simulink model "Control_with_duty"  (R2021a)
settings: Solver=VariableStepAuto  StartTime=0.0  StopTime=10  RelTol=1e-3
values from neighbouring files (symbols this model uses):
  Calc_delay = 20e-6    (= 2e-05)    [Control.m]
  J = 0.00052*1000    (= 0.52)    [Control.m]
  Kf = 0.1*10    (= 1)    [Control.m]
  Ki = double(vpasolve(num(3)==Ki/Lq,Ki))    [Control.m]
  Kp = double(vpasolve(num(2)==Rq/Lq+Kp/Lq,Kp))    [Control.m]
  lambda = 0.032    [Control.m]
  Ld = Lq    (= 5.25e-05)    [Control.m]
  Lq = 0.0525*10^-3    (= 5.25e-05)    [Control.m]
  Rd = 0.013/2    (= 0.0065)    [Control.m]
  Rq = Rd    (= 0.0065)    [Control.m]
  Ts = 1/Fsw    (= 9.3808630394e-05)    [Control.m]
  Vbat = 14.4*4    (= 57.6)    [Control.m]
libraries: mcbcontrolslib x6
settings Model: Creator=jacob  LastModifiedBy=jacob

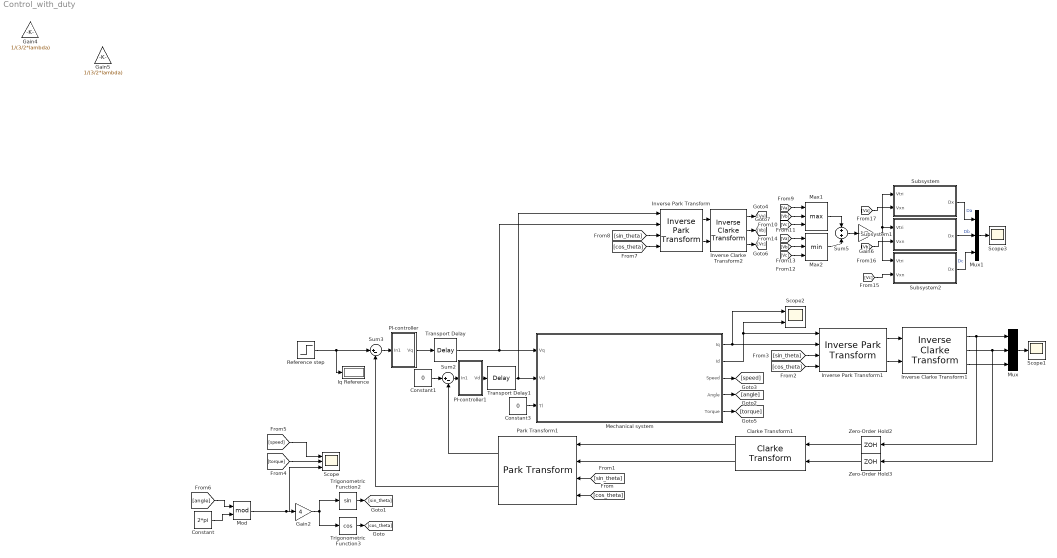
== system Control_with_duty ==
  Clarke Transform1 : mcbcontrolslib/Clarke Transform  VariantControl=Variant2
  Constant : Constant  Value=2*pi
  Constant1 : Constant  Value=0
  Constant3 : Constant  Value=0
  Gain2 : Gain  Gain=4
  Gain4 : Gain  Gain=1/(3/2*lambda)
  Gain5 : Gain  Gain=1/(3/2*lambda)
  Gain6 : Gain  Gain=-1/2
  Inverse Clarke Transform1 : mcbcontrolslib/Inverse Clarke Transform
      settings: SourceProductBaseCode=MT
  Inverse Clarke Transform2 : mcbcontrolslib/Inverse Clarke Transform
      settings: SourceProductBaseCode=MT
  Inverse Park Transform : mcbcontrolslib/Inverse Park Transform  AxisAlignment=D-axis
  Inverse Park Transform1 : mcbcontrolslib/Inverse Park Transform  AxisAlignment=D-axis
  Iq Reference : Display
      settings: Decimation=3
  Max1 : MinMax  Function=max  Inputs=3
  Max2 : MinMax  Inputs=3
  Mechanical system : Subsystem
  Mod : Math  Operator=mod  SaturateOnIntegerOverflow=on
  Mux : Mux  Inputs=3
  Mux1 : Mux  Inputs=3
  PI-controller : Subsystem
  PI-controller1 : Subsystem
  Park Transform1 : mcbcontrolslib/Park Transform  AxisAlignment=D-axis
      settings: SourceProductBaseCode=MT
  Reference step : Step  Time=0.1  After=311  SampleTime=0
  Scope : Scope  NumInputPorts=3
  Scope1 : Scope
  Scope2 : Scope  NumInputPorts=2
  Scope3 : Scope
  Subsystem : Subsystem
  Subsystem1 : Subsystem
  Subsystem2 : Subsystem
  Sum2 : Sum  Inputs=|+-
  Sum3 : Sum  Inputs=|+-
  Sum5 : Sum  Inputs=+|+
  Transport Delay : TransportDelay  DelayTime=Calc_delay
  Transport Delay1 : TransportDelay  DelayTime=Calc_delay
  Trigonometric Function2 : Trigonometry
  Trigonometric Function3 : Trigonometry  Operator=cos
  Zero-Order Hold2 : ZeroOrderHold  SampleTime=Ts
  Zero-Order Hold3 : ZeroOrderHold  SampleTime=Ts
  wires:
  Sum2/1 -> PI-controller1/1(In1)
  Inverse Park Transform1/2 -> Inverse Clarke Transform1/2
  [torque] -> Scope/2
  [sin_theta] -> Inverse Park Transform1/3
  [angle] -> Mod/1
  Constant/1 -> Mod/2
  Reference step/1 -> Sum3/1, Iq Reference/1
  Clarke Transform1/1 -> Park Transform1/1
  Clarke Transform1/2 -> Park Transform1/2
  Inverse Clarke Transform1/2 -> Zero-Order Hold3/1, Mux/2
  Inverse Park Transform1/1 -> Inverse Clarke Transform1/1
  Gain2/1 -> Trigonometric Function3/1, Trigonometric Function2/1
  Mux/1 -> Scope1/1
  Mechanical system/5(Torque) -> [torque]
  Sum3/1 -> PI-controller/1(In1)
  Inverse Clarke Transform1/3 -> Mux/3
  Park Transform1/1 -> Sum2/2
  Trigonometric Function3/1 -> [cos_theta]
  PI-controller1/1(Vd) -> Transport Delay1/1
  Mechanical system/1(Iq) -> Inverse Park Transform1/2, Scope2/1
  Inverse Clarke Transform1/1 -> Zero-Order Hold2/1, Mux/1
  Mechanical system/4(Angle) -> [angle]
  Mechanical system/2(Id) -> Inverse Park Transform1/1, Scope2/2
  Park Transform1/2 -> Sum3/2
  [cos_theta] -> Park Transform1/4
  [cos_theta] -> Inverse Park Transform1/4
  Constant3/1 -> Mechanical system/3(Tl)
  Mechanical system/3(Speed) -> [speed]
  Constant1/1 -> Sum2/1
  Zero-Order Hold3/1 -> Clarke Transform1/2
  [speed] -> Scope/1
  Mod/1 -> Scope/3, Gain2/1
  [sin_theta] -> Park Transform1/3
  PI-controller/1(Vq) -> Transport Delay/1
  Trigonometric Function2/1 -> [sin_theta]
  Zero-Order Hold2/1 -> Clarke Transform1/1
  Inverse Park Transform/1 -> Inverse Clarke Transform2/1
  Inverse Park Transform/2 -> Inverse Clarke Transform2/2
  [cos_theta] -> Inverse Park Transform/4
  [sin_theta] -> Inverse Park Transform/3
  Mux1/1 -> Scope3/1
  Subsystem/1(Dx) -> Mux1/1  "Da"
  Transport Delay1/1 -> Mechanical system/2(Vd), Inverse Park Transform/1
  Transport Delay/1 -> Inverse Park Transform/2, Mechanical system/1(Vq)
  Max2/1 -> Sum5/2
  Sum5/1 -> Gain6/1
  Max1/1 -> Sum5/1
  Inverse Clarke Transform2/1 -> [Va]
  Inverse Clarke Transform2/2 -> [Vb]
  Inverse Clarke Transform2/3 -> [Vc]
  Gain6/1 -> Subsystem1/1(Vtri), Subsystem/1(Vtri), Subsystem2/1(Vtri)
  [Va] -> Max2/1
  [Vb] -> Max2/2
  [Vc] -> Max2/3
  [Va] -> Max1/1
  [Vb] -> Max1/2
  [Vc] -> Max1/3
  [Va] -> Subsystem/2(Vxn)
  [Vc] -> Subsystem2/2(Vxn)
  [Vb] -> Subsystem1/2(Vxn)
  Subsystem2/1(Dx) -> Mux1/3  "Dc"
  Subsystem1/1(Dx) -> Mux1/2  "Db"

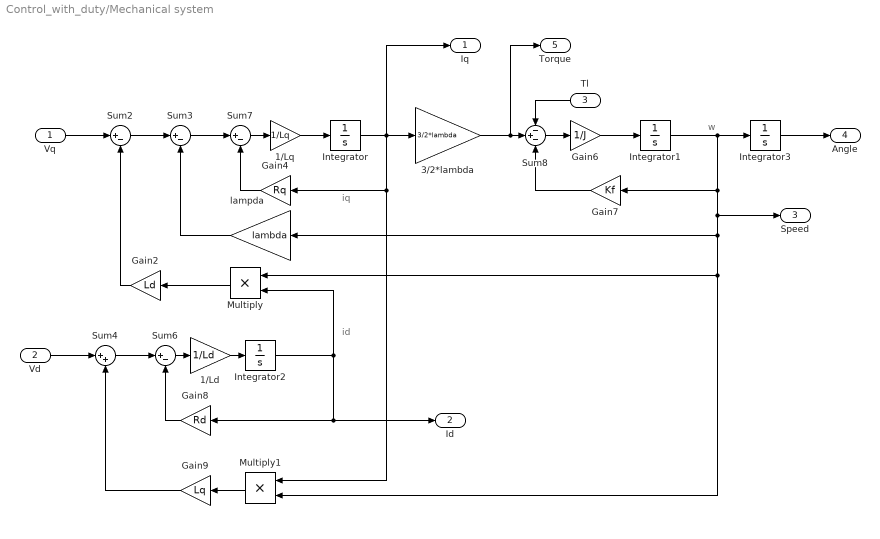
== system Control_with_duty/Mechanical system ==
  note: iq
  note: w
  note: id
  Vq : Inport
  Vd : Inport  Port=2
  Tl : Inport  Port=3
  1/Ld : Gain  Gain=1/Ld
  1/Lq : Gain  Gain=1/Lq
  3/2*lambda : Gain  Gain=3/2*lambda
  Gain2 : Gain  Gain=Ld
  Gain4 : Gain  Gain=Rq
  Gain6 : Gain  Gain=1/J
  Gain7 : Gain  Gain=Kf
  Gain8 : Gain  Gain=Rd
  Gain9 : Gain  Gain=Lq
  Integrator{,1..3} (4 alike) : Integrator
  Multiply : Product
  Multiply1 : Product
  Sum{2..3,6..7} (4 alike) : Sum  Inputs=|+-
  Sum4 : Sum  Inputs=|++
  Sum8 : Sum  Inputs=-+-
  lampda : Gain  Gain=lambda
  Iq : Outport
  Id : Outport  Port=2
  Speed : Outport  Port=3
  Angle : Outport  Port=4
  Torque : Outport  Port=5
  wires:
  Gain4/1 -> Sum7/2
  Sum2/1 -> Sum3/1
  Gain6/1 -> Integrator1/1
  Sum7/1 -> 1/Lq/1
  Vd/1 -> Sum4/1
  Sum6/1 -> 1/Ld/1
  Sum4/1 -> Sum6/1
  lampda/1 -> Sum3/2
  1/Lq/1 -> Integrator/1
  Gain2/1 -> Sum2/2
  Integrator2/1 -> Id/1, Gain8/1, Multiply/2
  Integrator1/1 -> Integrator3/1, Speed/1, Multiply1/2, Multiply/1, lampda/1, Gain7/1
  Sum8/1 -> Gain6/1
  Integrator/1 -> 3/2*lambda/1, Gain4/1, Multiply1/1, Iq/1
  Integrator3/1 -> Angle/1
  Multiply1/1 -> Gain9/1
  Gain9/1 -> Sum4/2
  Gain8/1 -> Sum6/2
  1/Ld/1 -> Integrator2/1
  Sum3/1 -> Sum7/1
  Multiply/1 -> Gain2/1
  Vq/1 -> Sum2/1
  3/2*lambda/1 -> Sum8/2, Torque/1
  Gain7/1 -> Sum8/3
  Tl/1 -> Sum8/1

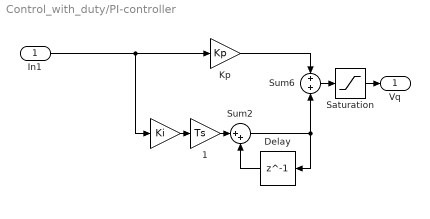
== system Control_with_duty/PI-controller ==
  In1 : Inport
  " " : Gain  Gain=Ki
  " 1" : Gain  Gain=Ts
  Delay : Delay  DelayLength=1  SampleTime=Ts
  Kp : Gain  Gain=Kp
  Saturation : Saturate  UpperLimit=Vbat  LowerLimit=-Vbat
  Sum2 : Sum  Inputs=|++
  Sum6 : Sum  Inputs=+|+
  Vq : Outport
  wires:
  " 1"/1 -> Sum2/1
  Delay/1 -> Sum2/2
  Kp/1 -> Sum6/1
  " "/1 -> " 1"/1
  Sum2/1 -> Delay/1, Sum6/2
  In1/1 -> " "/1, Kp/1
  Sum6/1 -> Saturation/1
  Saturation/1 -> Vq/1

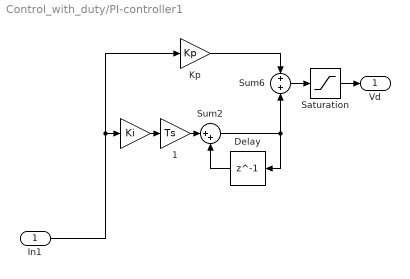
== system Control_with_duty/PI-controller1 ==
  In1 : Inport
  " " : Gain  Gain=Ki
  " 1" : Gain  Gain=Ts
  Delay : Delay  DelayLength=1  SampleTime=Ts
  Kp : Gain  Gain=Kp
  Saturation : Saturate  UpperLimit=Vbat  LowerLimit=-Vbat
  Sum2 : Sum  Inputs=|++
  Sum6 : Sum  Inputs=+|+
  Vd : Outport
  wires:
  " 1"/1 -> Sum2/1
  Delay/1 -> Sum2/2
  Kp/1 -> Sum6/1
  " "/1 -> " 1"/1
  Sum2/1 -> Delay/1, Sum6/2
  In1/1 -> Kp/1, " "/1
  Saturation/1 -> Vd/1
  Sum6/1 -> Saturation/1

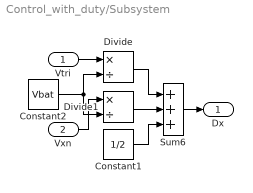
== system Control_with_duty/Subsystem ==
  Vtri : Inport
  Vxn : Inport  Port=2
  Constant1 : Constant  Value=1/2
  Constant2 : Constant  Value=Vbat
  Divide : Product  Inputs=*/
  Divide1 : Product  Inputs=*/
  Sum6 : Sum  Inputs=+++
  Dx : Outport
  wires:
  Vxn/1 -> Divide1/1
  Divide1/1 -> Sum6/2
  Constant1/1 -> Sum6/3
  Vtri/1 -> Divide/1
  Constant2/1 -> Divide/2, Divide1/2
  Sum6/1 -> Dx/1
  Divide/1 -> Sum6/1

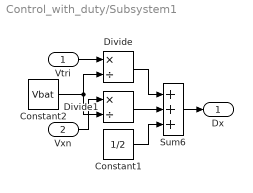
== system Control_with_duty/Subsystem1 ==
  Vtri : Inport
  Vxn : Inport  Port=2
  Constant1 : Constant  Value=1/2
  Constant2 : Constant  Value=Vbat
  Divide : Product  Inputs=*/
  Divide1 : Product  Inputs=*/
  Sum6 : Sum  Inputs=+++
  Dx : Outport
  wires:
  Divide/1 -> Sum6/1
  Constant2/1 -> Divide/2, Divide1/2
  Divide1/1 -> Sum6/2
  Vtri/1 -> Divide/1
  Vxn/1 -> Divide1/1
  Constant1/1 -> Sum6/3
  Sum6/1 -> Dx/1

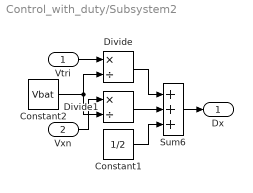
== system Control_with_duty/Subsystem2 ==
  Vtri : Inport
  Vxn : Inport  Port=2
  Constant1 : Constant  Value=1/2
  Constant2 : Constant  Value=Vbat
  Divide : Product  Inputs=*/
  Divide1 : Product  Inputs=*/
  Sum6 : Sum  Inputs=+++
  Dx : Outport
  wires:
  Divide/1 -> Sum6/1
  Constant2/1 -> Divide/2, Divide1/2
  Divide1/1 -> Sum6/2
  Vtri/1 -> Divide/1
  Vxn/1 -> Divide1/1
  Constant1/1 -> Sum6/3
  Sum6/1 -> Dx/1
